simulink library "Si_block"  (R2023a)
settings: Solver=VariableStepAuto  StartTime=0.0  StopTime=10.0  RelTol=1e-3
values from neighbouring files (symbols this model uses):
  A = A_contr    [coop_reg.m]
  Adj = zeros(N,N)    [main.m]    (also in network_config.m)
  B = [0 -9.9453]'    [coop_reg.m]
  C = [708.27 0]    [coop_reg.m]
  c = par.c_fact * c_min    [coop_reg.m]
  co = par.co_fact * c_min    [coop_reg.m]
  D = 0    [coop_reg.m]
  F = L_obs / c    [coop_reg.m]
  g = zeros(N,1)    [main.m]    (also in network_config.m)
  K = inv(R)*B'*P    [coop_reg.m]
  local_obs = false    [main.m]
  noise_mean = 0    [coop_reg.m]
  noise_seed = randi(1000)    [coop_reg.m]
  noise_var = 100    [coop_reg.m]
  noise_vec = zeros(N+1,1)    [CPS_sim.m]    (also in coop_reg.m = noise_vec(1:N); main.m)
  xi_0 = [0 0]    [coop_reg.m]
  xi_0_obs = zeros(n,1)    [coop_reg.m]
undefined symbols (not defined in the file or in its folder): gen_coopObserver
settings Model: Creator=Francesco  LastModifiedBy=federico
settings RTWCC: GPUComputeCapability=5.0

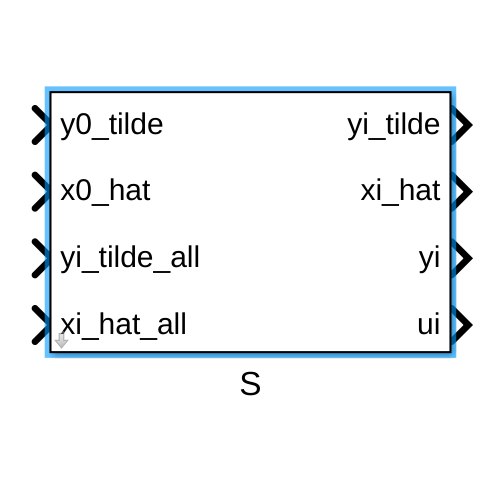
[thumbnail: Simulink's stored preview of the top-level diagram]
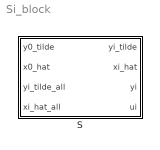
== system Si_block ==
  S : Subsystem  mask{i=0}
      mask prompts: i "Agent index"

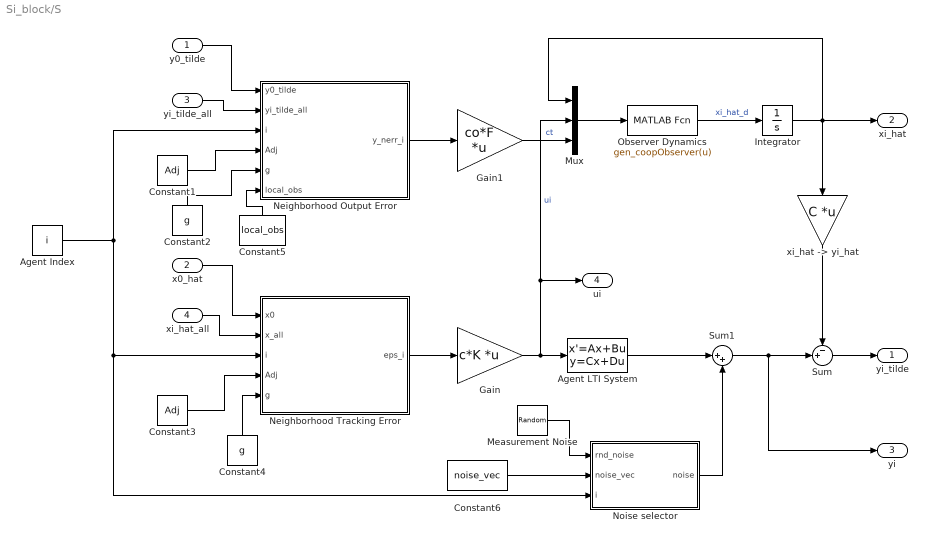
== system Si_block/S ==
  y0_tilde : Inport
  x0_hat : Inport  Port=2
  yi_tilde_all : Inport  Port=3
  xi_hat_all : Inport  Port=4
  Agent Index : Constant  Value=i
  Agent LTI System : StateSpace  A=A  B=B  C=C  D=D  InitialCondition=xi_0
  Constant1 : Constant  Value=Adj
  Constant2 : Constant  Value=g
  Constant3 : Constant  Value=Adj
  Constant4 : Constant  Value=g
  Constant5 : Constant  Value=local_obs
  Constant6 : Constant  Value=noise_vec
  Gain : Gain  Gain=c*K  Multiplication=Matrix(K*u)
  Gain1 : Gain  Gain=co*F  Multiplication=Matrix(K*u)
  Integrator : Integrator  InitialCondition=xi_0_obs
  Measurement Noise : RandomNumber  Mean=noise_mean  Variance=noise_var  Seed=noise_seed  SampleTime=0.1
  Mux : Mux  Inputs=3
  Neighborhood Output Error : MATLAB Function  TreatAsAtomicUnit=on
  Neighborhood Tracking Error : MATLAB Function  TreatAsAtomicUnit=on
  Noise selector : MATLAB Function  TreatAsAtomicUnit=on
  Observer Dynamics : MATLABFcn  MATLABFcn=gen_coopObserver(u)
  Sum : Sum  Inputs=-+|
  Sum1 : Sum  Inputs=|++
  "xi_hat -> yi_hat" : Gain  Gain=C  Multiplication=Matrix(K*u)
  yi_tilde : Outport
  xi_hat : Outport  Port=2
  yi : Outport  Port=3
  ui : Outport  Port=4
  wires:
  Gain/1 -> ui/1, Mux/2, Agent LTI System/1  "ui"
  Neighborhood Tracking Error/1(eps_i) -> Gain/1
  Neighborhood Output Error/1(y_nerr_i) -> Gain1/1
  Gain1/1 -> Mux/3  "ct"
  Mux/1 -> Observer Dynamics/1
  Observer Dynamics/1 -> Integrator/1  "xi_hat_d"
  Integrator/1 -> Mux/1, "xi_hat -> yi_hat"/1, xi_hat/1
  y0_tilde/1 -> Neighborhood Output Error/1(y0_tilde)
  yi_tilde_all/1 -> Neighborhood Output Error/2(yi_tilde_all)
  x0_hat/1 -> Neighborhood Tracking Error/1(x0)
  xi_hat_all/1 -> Neighborhood Tracking Error/2(x_all)
  Constant1/1 -> Neighborhood Output Error/4(Adj)
  Constant2/1 -> Neighborhood Output Error/5(g)
  Agent Index/1 -> Neighborhood Output Error/3(i), Noise selector/3(i), Neighborhood Tracking Error/3(i)
  Constant3/1 -> Neighborhood Tracking Error/4(Adj)
  Constant4/1 -> Neighborhood Tracking Error/5(g)
  "xi_hat -> yi_hat"/1 -> Sum/1
  Sum/1 -> yi_tilde/1
  Constant5/1 -> Neighborhood Output Error/6(local_obs)
  Agent LTI System/1 -> Sum1/1
  Sum1/1 -> yi/1, Sum/2
  Measurement Noise/1 -> Noise selector/1(rnd_noise)
  Constant6/1 -> Noise selector/2(noise_vec)
  Noise selector/1(noise) -> Sum1/2

== matlab function Si_block/S/Neighborhood Output Error ==
  data: y0_tilde input; yi_tilde_all input; y_nerr_i output; i input; Adj input; g input; local_obs input
function y_nerr_i = fcn(y0_tilde, yi_tilde_all, i, Adj, g, local_obs)

N = 6;
n = 2;
p = 1;

yi_tilde_all = reshape(yi_tilde_all, [p,N]);

y_nerr_i = zeros(p,1);
for j = 1:size(Adj,1)
    y_nerr_i = y_nerr_i + Adj(i,j) * (yi_tilde_all(:,j) - yi_tilde_all(:,i));
end
y_nerr_i = y_nerr_i + g(i) * (y0_tilde - yi_tilde_all(:,i));

if local_obs
    y_nerr_i = yi_tilde_all(:,i);
end

== matlab function Si_block/S/Neighborhood Tracking Error ==
  data: x0 input; x_all input; eps_i output; i input; Adj input; g input
function eps_i = fcn(x0, x_all, i, Adj, g)

N = 6;
n = 2;

x_all = reshape(x_all, [n,N]);

eps_i = zeros(n,1);
for j = 1:size(Adj,1)
    eps_i = eps_i + Adj(i,j) * (x_all(:,j) - x_all(:,i));
end
eps_i = eps_i + g(i) * (x0 - x_all(:,i));

== matlab function Si_block/S/Noise selector ==
  data: rnd_noise input; noise output; noise_vec input; i input
function noise = fcn(rnd_noise, noise_vec, i)

noise = rnd_noise * noise_vec(i);
